simulink model "Sim"  (R2016a)
settings: Solver=VariableStepAuto  StartTime=0.0  StopTime=1500  FixedStep=1  RelTol=1e-3
values from neighbouring files (symbols this model uses):
  A = 7.841E16    (= 7.841e+16)    [Parameters.m]
  cv = 1820000    [Parameters.m]
  detaX = 0.0013333    [Parameters.m]
  Ea = 1.4766E5    (= 147660)    [Parameters.m]
  H_dr = 4.92E8    (= 492000000)    [Parameters.m]
  H_pc = 1.992E8    (= 199200000)    [Parameters.m]
  ord = 0.75    [Parameters.m]
  q_dot = 3.981E4    (= 39810)    [Parameters.m]
  T_0 = 298.15    [Parameters.m]
  Tl = 334.15    [Parameters.m]
  Ts = 331.15    [Parameters.m]
(part 2 of 3)

== system Sim/Element27 ==
  Q_in : Inport
  Q_out : Inport  Port=2
  Add : Sum  Inputs=++-
  Bias : Bias  Bias=1
  Bias2 : Bias  Bias=-Ts
  Bias3 : Bias  Bias=-Tl
  Bias4 : Bias  Bias=-1
  Constant : Constant  Value=cv+(H_pc/(Tl-Ts))
  Constant1 : Constant  Value=cv
  Constant2 : Constant  Value=0
  Constant3 : Constant  Value=ord
  Constant4 : Constant
  Divide : Product  Inputs=/
  Divide1 : Product  Inputs=/*
  Gain : Gain  Gain=-1
  Gain1 : Gain  Gain=(-8.314)/Ea
  Gain2 : Gain  Gain=(-1)*H_dr*A
  Gain3 : Gain  Gain=-1
  Gain4 : Gain  Gain=(-1)/H_dr
  Gain5 : Gain  Gain=1/(Tl-Ts)
  Gain6 : Gain  Gain=-1
  Integrator : Integrator  InitialCondition=T_0
  Integrator1 : Integrator
  Math Function : Math  SaturateOnIntegerOverflow=on
  Math Function1 : Math  Operator=pow  SaturateOnIntegerOverflow=on
  Product : Product
  Switch : Switch
  Switch1 : Switch  Criteria=u2 > Threshold
  Switch2 : Switch
  Switch3 : Switch  Criteria=u2 > Threshold
  Beta : Outport
  Temp : Outport  Port=2
  Alpha : Outport  Port=3
  wires:
  Q_out/1 -> Add/3
  Gain/1 -> Bias/1
  Divide1/1 -> Integrator/1  "dT/dt"
  Gain2/1 -> Product/1
  Integrator/1 -> Temp/1, Bias3/1, Bias2/1, Gain1/1  "T"
  Switch1/1 -> Divide1/1  "CON"
  Math Function1/1 -> Product/2
  Bias/1 -> Math Function1/1  "(1-Alpha)"
  Constant2/1 -> Switch2/3
  Add/1 -> Divide1/2  "CON*(dT/dt)"
  Gain5/1 -> Switch2/1, Switch2/2
  Switch2/1 -> Switch3/1, Bias4/1
  Constant/1 -> Switch/1
  Bias4/1 -> Gain6/1
  Switch/1 -> Switch1/1
  Switch3/1 -> Beta/1  "Beta"
  Gain6/1 -> Switch3/2
  Bias2/1 -> Gain5/1, Switch/2
  Constant4/1 -> Switch3/3
  Product/1 -> Add/1, Gain4/1  "-A*H_dr*exp()*(-Alhpa)"
  Gain1/1 -> Divide/1  "(-R*T)/Ea"
  Integrator1/1 -> Gain/1, Alpha/1  "Alpha"
  Gain4/1 -> Integrator1/1
  Constant3/1 -> Math Function1/2
  Constant1/1 -> Switch/3, Switch1/3
  Divide/1 -> Math Function/1  "Ea/(-R*T)"
  Math Function/1 -> Gain2/1
  Bias3/1 -> Gain3/1
  Gain3/1 -> Switch1/2
  Q_in/1 -> Add/2

== system Sim/Element28 ==
  Q_in : Inport
  Q_out : Inport  Port=2
  Add : Sum  Inputs=++-
  Bias : Bias  Bias=1
  Bias2 : Bias  Bias=-Ts
  Bias3 : Bias  Bias=-Tl
  Bias4 : Bias  Bias=-1
  Constant : Constant  Value=cv+(H_pc/(Tl-Ts))
  Constant1 : Constant  Value=cv
  Constant2 : Constant  Value=0
  Constant3 : Constant  Value=ord
  Constant4 : Constant
  Divide : Product  Inputs=/
  Divide1 : Product  Inputs=/*
  Gain : Gain  Gain=-1
  Gain1 : Gain  Gain=(-8.314)/Ea
  Gain2 : Gain  Gain=(-1)*H_dr*A
  Gain3 : Gain  Gain=-1
  Gain4 : Gain  Gain=(-1)/H_dr
  Gain5 : Gain  Gain=1/(Tl-Ts)
  Gain6 : Gain  Gain=-1
  Integrator : Integrator  InitialCondition=T_0
  Integrator1 : Integrator
  Math Function : Math  SaturateOnIntegerOverflow=on
  Math Function1 : Math  Operator=pow  SaturateOnIntegerOverflow=on
  Product : Product
  Switch : Switch
  Switch1 : Switch  Criteria=u2 > Threshold
  Switch2 : Switch
  Switch3 : Switch  Criteria=u2 > Threshold
  Beta : Outport
  Temp : Outport  Port=2
  Alpha : Outport  Port=3
  wires:
  Q_out/1 -> Add/3
  Gain/1 -> Bias/1
  Divide1/1 -> Integrator/1  "dT/dt"
  Gain2/1 -> Product/1
  Integrator/1 -> Temp/1, Bias3/1, Bias2/1, Gain1/1  "T"
  Switch1/1 -> Divide1/1  "CON"
  Math Function1/1 -> Product/2
  Bias/1 -> Math Function1/1  "(1-Alpha)"
  Constant2/1 -> Switch2/3
  Add/1 -> Divide1/2  "CON*(dT/dt)"
  Gain5/1 -> Switch2/1, Switch2/2
  Switch2/1 -> Switch3/1, Bias4/1
  Constant/1 -> Switch/1
  Bias4/1 -> Gain6/1
  Switch/1 -> Switch1/1
  Switch3/1 -> Beta/1  "Beta"
  Gain6/1 -> Switch3/2
  Bias2/1 -> Gain5/1, Switch/2
  Constant4/1 -> Switch3/3
  Product/1 -> Add/1, Gain4/1  "-A*H_dr*exp()*(-Alhpa)"
  Gain1/1 -> Divide/1  "(-R*T)/Ea"
  Integrator1/1 -> Gain/1, Alpha/1  "Alpha"
  Gain4/1 -> Integrator1/1
  Constant3/1 -> Math Function1/2
  Constant1/1 -> Switch/3, Switch1/3
  Divide/1 -> Math Function/1  "Ea/(-R*T)"
  Math Function/1 -> Gain2/1
  Bias3/1 -> Gain3/1
  Gain3/1 -> Switch1/2
  Q_in/1 -> Add/2

== system Sim/Element29 ==
  Q_in : Inport
  Q_out : Inport  Port=2
  Add : Sum  Inputs=++-
  Bias : Bias  Bias=1
  Bias2 : Bias  Bias=-Ts
  Bias3 : Bias  Bias=-Tl
  Bias4 : Bias  Bias=-1
  Constant : Constant  Value=cv+(H_pc/(Tl-Ts))
  Constant1 : Constant  Value=cv
  Constant2 : Constant  Value=0
  Constant3 : Constant  Value=ord
  Constant4 : Constant
  Divide : Product  Inputs=/
  Divide1 : Product  Inputs=/*
  Gain : Gain  Gain=-1
  Gain1 : Gain  Gain=(-8.314)/Ea
  Gain2 : Gain  Gain=(-1)*H_dr*A
  Gain3 : Gain  Gain=-1
  Gain4 : Gain  Gain=(-1)/H_dr
  Gain5 : Gain  Gain=1/(Tl-Ts)
  Gain6 : Gain  Gain=-1
  Integrator : Integrator  InitialCondition=T_0
  Integrator1 : Integrator
  Math Function : Math  SaturateOnIntegerOverflow=on
  Math Function1 : Math  Operator=pow  SaturateOnIntegerOverflow=on
  Product : Product
  Switch : Switch
  Switch1 : Switch  Criteria=u2 > Threshold
  Switch2 : Switch
  Switch3 : Switch  Criteria=u2 > Threshold
  Beta : Outport
  Temp : Outport  Port=2
  Alpha : Outport  Port=3
  wires:
  Q_out/1 -> Add/3
  Gain/1 -> Bias/1
  Divide1/1 -> Integrator/1  "dT/dt"
  Gain2/1 -> Product/1
  Integrator/1 -> Temp/1, Bias3/1, Bias2/1, Gain1/1  "T"
  Switch1/1 -> Divide1/1  "CON"
  Math Function1/1 -> Product/2
  Bias/1 -> Math Function1/1  "(1-Alpha)"
  Constant2/1 -> Switch2/3
  Add/1 -> Divide1/2  "CON*(dT/dt)"
  Gain5/1 -> Switch2/1, Switch2/2
  Switch2/1 -> Switch3/1, Bias4/1
  Constant/1 -> Switch/1
  Bias4/1 -> Gain6/1
  Switch/1 -> Switch1/1
  Switch3/1 -> Beta/1  "Beta"
  Gain6/1 -> Switch3/2
  Bias2/1 -> Gain5/1, Switch/2
  Constant4/1 -> Switch3/3
  Product/1 -> Add/1, Gain4/1  "-A*H_dr*exp()*(-Alhpa)"
  Gain1/1 -> Divide/1  "(-R*T)/Ea"
  Integrator1/1 -> Gain/1, Alpha/1  "Alpha"
  Gain4/1 -> Integrator1/1
  Constant3/1 -> Math Function1/2
  Constant1/1 -> Switch/3, Switch1/3
  Divide/1 -> Math Function/1  "Ea/(-R*T)"
  Math Function/1 -> Gain2/1
  Bias3/1 -> Gain3/1
  Gain3/1 -> Switch1/2
  Q_in/1 -> Add/2

== system Sim/Element3 ==
  Q_in : Inport
  Q_out : Inport  Port=2
  Add : Sum  Inputs=++-
  Bias : Bias  Bias=1
  Bias2 : Bias  Bias=-Ts
  Bias3 : Bias  Bias=-Tl
  Bias4 : Bias  Bias=-1
  Constant : Constant  Value=cv+(H_pc/(Tl-Ts))
  Constant1 : Constant  Value=cv
  Constant2 : Constant  Value=0
  Constant3 : Constant  Value=ord
  Constant4 : Constant
  Divide : Product  Inputs=/
  Divide1 : Product  Inputs=/*
  Gain : Gain  Gain=-1
  Gain1 : Gain  Gain=(-8.314)/Ea
  Gain2 : Gain  Gain=(-1)*H_dr*A
  Gain3 : Gain  Gain=-1
  Gain4 : Gain  Gain=(-1)/H_dr
  Gain5 : Gain  Gain=1/(Tl-Ts)
  Gain6 : Gain  Gain=-1
  Integrator : Integrator  InitialCondition=T_0
  Integrator1 : Integrator
  Math Function : Math  SaturateOnIntegerOverflow=on
  Math Function1 : Math  Operator=pow  SaturateOnIntegerOverflow=on
  Product : Product
  Switch : Switch
  Switch1 : Switch  Criteria=u2 > Threshold
  Switch2 : Switch
  Switch3 : Switch  Criteria=u2 > Threshold
  Beta : Outport
  Temp : Outport  Port=2
  Alpha : Outport  Port=3
  wires:
  Q_out/1 -> Add/3
  Gain/1 -> Bias/1
  Divide1/1 -> Integrator/1  "dT/dt"
  Gain2/1 -> Product/1
  Integrator/1 -> Temp/1, Bias3/1, Bias2/1, Gain1/1  "T"
  Switch1/1 -> Divide1/1  "CON"
  Math Function1/1 -> Product/2
  Bias/1 -> Math Function1/1  "(1-Alpha)"
  Constant2/1 -> Switch2/3
  Add/1 -> Divide1/2  "CON*(dT/dt)"
  Gain5/1 -> Switch2/1, Switch2/2
  Switch2/1 -> Switch3/1, Bias4/1
  Constant/1 -> Switch/1
  Bias4/1 -> Gain6/1
  Switch/1 -> Switch1/1
  Switch3/1 -> Beta/1  "Beta"
  Gain6/1 -> Switch3/2
  Bias2/1 -> Gain5/1, Switch/2
  Constant4/1 -> Switch3/3
  Product/1 -> Add/1, Gain4/1  "-A*H_dr*exp()*(-Alhpa)"
  Gain1/1 -> Divide/1  "(-R*T)/Ea"
  Integrator1/1 -> Gain/1, Alpha/1  "Alpha"
  Gain4/1 -> Integrator1/1
  Constant3/1 -> Math Function1/2
  Constant1/1 -> Switch/3, Switch1/3
  Divide/1 -> Math Function/1  "Ea/(-R*T)"
  Math Function/1 -> Gain2/1
  Bias3/1 -> Gain3/1
  Gain3/1 -> Switch1/2
  Q_in/1 -> Add/2

== system Sim/Element30 ==
  Q_in : Inport
  Q_out : Inport  Port=2
  Add : Sum  Inputs=++-
  Bias : Bias  Bias=1
  Bias2 : Bias  Bias=-Ts
  Bias3 : Bias  Bias=-Tl
  Bias4 : Bias  Bias=-1
  Constant : Constant  Value=cv+(H_pc/(Tl-Ts))
  Constant1 : Constant  Value=cv
  Constant2 : Constant  Value=0
  Constant3 : Constant  Value=ord
  Constant4 : Constant
  Divide : Product  Inputs=/
  Divide1 : Product  Inputs=/*
  Gain : Gain  Gain=-1
  Gain1 : Gain  Gain=(-8.314)/Ea
  Gain2 : Gain  Gain=(-1)*H_dr*A
  Gain3 : Gain  Gain=-1
  Gain4 : Gain  Gain=(-1)/H_dr
  Gain5 : Gain  Gain=1/(Tl-Ts)
  Gain6 : Gain  Gain=-1
  Integrator : Integrator  InitialCondition=T_0
  Integrator1 : Integrator
  Math Function : Math  SaturateOnIntegerOverflow=on
  Math Function1 : Math  Operator=pow  SaturateOnIntegerOverflow=on
  Product : Product
  Switch : Switch
  Switch1 : Switch  Criteria=u2 > Threshold
  Switch2 : Switch
  Switch3 : Switch  Criteria=u2 > Threshold
  Beta : Outport
  Temp : Outport  Port=2
  Alpha : Outport  Port=3
  wires:
  Q_out/1 -> Add/3
  Gain/1 -> Bias/1
  Divide1/1 -> Integrator/1  "dT/dt"
  Gain2/1 -> Product/1
  Integrator/1 -> Temp/1, Bias3/1, Bias2/1, Gain1/1  "T"
  Switch1/1 -> Divide1/1  "CON"
  Math Function1/1 -> Product/2
  Bias/1 -> Math Function1/1  "(1-Alpha)"
  Constant2/1 -> Switch2/3
  Add/1 -> Divide1/2  "CON*(dT/dt)"
  Gain5/1 -> Switch2/1, Switch2/2
  Switch2/1 -> Switch3/1, Bias4/1
  Constant/1 -> Switch/1
  Bias4/1 -> Gain6/1
  Switch/1 -> Switch1/1
  Switch3/1 -> Beta/1  "Beta"
  Gain6/1 -> Switch3/2
  Bias2/1 -> Gain5/1, Switch/2
  Constant4/1 -> Switch3/3
  Product/1 -> Add/1, Gain4/1  "-A*H_dr*exp()*(-Alhpa)"
  Gain1/1 -> Divide/1  "(-R*T)/Ea"
  Integrator1/1 -> Gain/1, Alpha/1  "Alpha"
  Gain4/1 -> Integrator1/1
  Constant3/1 -> Math Function1/2
  Constant1/1 -> Switch/3, Switch1/3
  Divide/1 -> Math Function/1  "Ea/(-R*T)"
  Math Function/1 -> Gain2/1
  Bias3/1 -> Gain3/1
  Gain3/1 -> Switch1/2
  Q_in/1 -> Add/2

== system Sim/Element31 ==
  Q_in : Inport
  Q_out : Inport  Port=2
  Add : Sum  Inputs=++-
  Bias : Bias  Bias=1
  Bias2 : Bias  Bias=-Ts
  Bias3 : Bias  Bias=-Tl
  Bias4 : Bias  Bias=-1
  Constant : Constant  Value=cv+(H_pc/(Tl-Ts))
  Constant1 : Constant  Value=cv
  Constant2 : Constant  Value=0
  Constant3 : Constant  Value=ord
  Constant4 : Constant
  Divide : Product  Inputs=/
  Divide1 : Product  Inputs=/*
  Gain : Gain  Gain=-1
  Gain1 : Gain  Gain=(-8.314)/Ea
  Gain2 : Gain  Gain=(-1)*H_dr*A
  Gain3 : Gain  Gain=-1
  Gain4 : Gain  Gain=(-1)/H_dr
  Gain5 : Gain  Gain=1/(Tl-Ts)
  Gain6 : Gain  Gain=-1
  Integrator : Integrator  InitialCondition=T_0
  Integrator1 : Integrator
  Math Function : Math  SaturateOnIntegerOverflow=on
  Math Function1 : Math  Operator=pow  SaturateOnIntegerOverflow=on
  Product : Product
  Switch : Switch
  Switch1 : Switch  Criteria=u2 > Threshold
  Switch2 : Switch
  Switch3 : Switch  Criteria=u2 > Threshold
  Beta : Outport
  Temp : Outport  Port=2
  Alpha : Outport  Port=3
  wires:
  Q_out/1 -> Add/3
  Gain/1 -> Bias/1
  Divide1/1 -> Integrator/1  "dT/dt"
  Gain2/1 -> Product/1
  Integrator/1 -> Temp/1, Bias3/1, Bias2/1, Gain1/1  "T"
  Switch1/1 -> Divide1/1  "CON"
  Math Function1/1 -> Product/2
  Bias/1 -> Math Function1/1  "(1-Alpha)"
  Constant2/1 -> Switch2/3
  Add/1 -> Divide1/2  "CON*(dT/dt)"
  Gain5/1 -> Switch2/1, Switch2/2
  Switch2/1 -> Switch3/1, Bias4/1
  Constant/1 -> Switch/1
  Bias4/1 -> Gain6/1
  Switch/1 -> Switch1/1
  Switch3/1 -> Beta/1  "Beta"
  Gain6/1 -> Switch3/2
  Bias2/1 -> Gain5/1, Switch/2
  Constant4/1 -> Switch3/3
  Product/1 -> Add/1, Gain4/1  "-A*H_dr*exp()*(-Alhpa)"
  Gain1/1 -> Divide/1  "(-R*T)/Ea"
  Integrator1/1 -> Gain/1, Alpha/1  "Alpha"
  Gain4/1 -> Integrator1/1
  Constant3/1 -> Math Function1/2
  Constant1/1 -> Switch/3, Switch1/3
  Divide/1 -> Math Function/1  "Ea/(-R*T)"
  Math Function/1 -> Gain2/1
  Bias3/1 -> Gain3/1
  Gain3/1 -> Switch1/2
  Q_in/1 -> Add/2

== system Sim/Element32 ==
  Q_in : Inport
  Q_out : Inport  Port=2
  Add : Sum  Inputs=++-
  Bias : Bias  Bias=1
  Bias2 : Bias  Bias=-Ts
  Bias3 : Bias  Bias=-Tl
  Bias4 : Bias  Bias=-1
  Constant : Constant  Value=cv+(H_pc/(Tl-Ts))
  Constant1 : Constant  Value=cv
  Constant2 : Constant  Value=0
  Constant3 : Constant  Value=ord
  Constant4 : Constant
  Divide : Product  Inputs=/
  Divide1 : Product  Inputs=/*
  Gain : Gain  Gain=-1
  Gain1 : Gain  Gain=(-8.314)/Ea
  Gain2 : Gain  Gain=(-1)*H_dr*A
  Gain3 : Gain  Gain=-1
  Gain4 : Gain  Gain=(-1)/H_dr
  Gain5 : Gain  Gain=1/(Tl-Ts)
  Gain6 : Gain  Gain=-1
  Integrator : Integrator  InitialCondition=T_0
  Integrator1 : Integrator
  Math Function : Math  SaturateOnIntegerOverflow=on
  Math Function1 : Math  Operator=pow  SaturateOnIntegerOverflow=on
  Product : Product
  Switch : Switch
  Switch1 : Switch  Criteria=u2 > Threshold
  Switch2 : Switch
  Switch3 : Switch  Criteria=u2 > Threshold
  Beta : Outport
  Temp : Outport  Port=2
  Alpha : Outport  Port=3
  wires:
  Q_out/1 -> Add/3
  Gain/1 -> Bias/1
  Divide1/1 -> Integrator/1  "dT/dt"
  Gain2/1 -> Product/1
  Integrator/1 -> Temp/1, Bias3/1, Bias2/1, Gain1/1  "T"
  Switch1/1 -> Divide1/1  "CON"
  Math Function1/1 -> Product/2
  Bias/1 -> Math Function1/1  "(1-Alpha)"
  Constant2/1 -> Switch2/3
  Add/1 -> Divide1/2  "CON*(dT/dt)"
  Gain5/1 -> Switch2/1, Switch2/2
  Switch2/1 -> Switch3/1, Bias4/1
  Constant/1 -> Switch/1
  Bias4/1 -> Gain6/1
  Switch/1 -> Switch1/1
  Switch3/1 -> Beta/1  "Beta"
  Gain6/1 -> Switch3/2
  Bias2/1 -> Gain5/1, Switch/2
  Constant4/1 -> Switch3/3
  Product/1 -> Add/1, Gain4/1  "-A*H_dr*exp()*(-Alhpa)"
  Gain1/1 -> Divide/1  "(-R*T)/Ea"
  Integrator1/1 -> Gain/1, Alpha/1  "Alpha"
  Gain4/1 -> Integrator1/1
  Constant3/1 -> Math Function1/2
  Constant1/1 -> Switch/3, Switch1/3
  Divide/1 -> Math Function/1  "Ea/(-R*T)"
  Math Function/1 -> Gain2/1
  Bias3/1 -> Gain3/1
  Gain3/1 -> Switch1/2
  Q_in/1 -> Add/2

== system Sim/Element33 ==
  Q_in : Inport
  Q_out : Inport  Port=2
  Add : Sum  Inputs=++-
  Bias : Bias  Bias=1
  Bias2 : Bias  Bias=-Ts
  Bias3 : Bias  Bias=-Tl
  Bias4 : Bias  Bias=-1
  Constant : Constant  Value=cv+(H_pc/(Tl-Ts))
  Constant1 : Constant  Value=cv
  Constant2 : Constant  Value=0
  Constant3 : Constant  Value=ord
  Constant4 : Constant
  Divide : Product  Inputs=/
  Divide1 : Product  Inputs=/*
  Gain : Gain  Gain=-1
  Gain1 : Gain  Gain=(-8.314)/Ea
  Gain2 : Gain  Gain=(-1)*H_dr*A
  Gain3 : Gain  Gain=-1
  Gain4 : Gain  Gain=(-1)/H_dr
  Gain5 : Gain  Gain=1/(Tl-Ts)
  Gain6 : Gain  Gain=-1
  Integrator : Integrator  InitialCondition=T_0
  Integrator1 : Integrator
  Math Function : Math  SaturateOnIntegerOverflow=on
  Math Function1 : Math  Operator=pow  SaturateOnIntegerOverflow=on
  Product : Product
  Switch : Switch
  Switch1 : Switch  Criteria=u2 > Threshold
  Switch2 : Switch
  Switch3 : Switch  Criteria=u2 > Threshold
  Beta : Outport
  Temp : Outport  Port=2
  Alpha : Outport  Port=3
  wires:
  Q_out/1 -> Add/3
  Gain/1 -> Bias/1
  Divide1/1 -> Integrator/1  "dT/dt"
  Gain2/1 -> Product/1
  Integrator/1 -> Temp/1, Bias3/1, Bias2/1, Gain1/1  "T"
  Switch1/1 -> Divide1/1  "CON"
  Math Function1/1 -> Product/2
  Bias/1 -> Math Function1/1  "(1-Alpha)"
  Constant2/1 -> Switch2/3
  Add/1 -> Divide1/2  "CON*(dT/dt)"
  Gain5/1 -> Switch2/1, Switch2/2
  Switch2/1 -> Switch3/1, Bias4/1
  Constant/1 -> Switch/1
  Bias4/1 -> Gain6/1
  Switch/1 -> Switch1/1
  Switch3/1 -> Beta/1  "Beta"
  Gain6/1 -> Switch3/2
  Bias2/1 -> Gain5/1, Switch/2
  Constant4/1 -> Switch3/3
  Product/1 -> Add/1, Gain4/1  "-A*H_dr*exp()*(-Alhpa)"
  Gain1/1 -> Divide/1  "(-R*T)/Ea"
  Integrator1/1 -> Gain/1, Alpha/1  "Alpha"
  Gain4/1 -> Integrator1/1
  Constant3/1 -> Math Function1/2
  Constant1/1 -> Switch/3, Switch1/3
  Divide/1 -> Math Function/1  "Ea/(-R*T)"
  Math Function/1 -> Gain2/1
  Bias3/1 -> Gain3/1
  Gain3/1 -> Switch1/2
  Q_in/1 -> Add/2

== system Sim/Element34 ==
  Q_in : Inport
  Q_out : Inport  Port=2
  Add : Sum  Inputs=++-
  Bias : Bias  Bias=1
  Bias2 : Bias  Bias=-Ts
  Bias3 : Bias  Bias=-Tl
  Bias4 : Bias  Bias=-1
  Constant : Constant  Value=cv+(H_pc/(Tl-Ts))
  Constant1 : Constant  Value=cv
  Constant2 : Constant  Value=0
  Constant3 : Constant  Value=ord
  Constant4 : Constant
  Divide : Product  Inputs=/
  Divide1 : Product  Inputs=/*
  Gain : Gain  Gain=-1
  Gain1 : Gain  Gain=(-8.314)/Ea
  Gain2 : Gain  Gain=(-1)*H_dr*A
  Gain3 : Gain  Gain=-1
  Gain4 : Gain  Gain=(-1)/H_dr
  Gain5 : Gain  Gain=1/(Tl-Ts)
  Gain6 : Gain  Gain=-1
  Integrator : Integrator  InitialCondition=T_0
  Integrator1 : Integrator
  Math Function : Math  SaturateOnIntegerOverflow=on
  Math Function1 : Math  Operator=pow  SaturateOnIntegerOverflow=on
  Product : Product
  Switch : Switch
  Switch1 : Switch  Criteria=u2 > Threshold
  Switch2 : Switch
  Switch3 : Switch  Criteria=u2 > Threshold
  Beta : Outport
  Temp : Outport  Port=2
  Alpha : Outport  Port=3
  wires:
  Q_out/1 -> Add/3
  Gain/1 -> Bias/1
  Divide1/1 -> Integrator/1  "dT/dt"
  Gain2/1 -> Product/1
  Integrator/1 -> Temp/1, Bias3/1, Bias2/1, Gain1/1  "T"
  Switch1/1 -> Divide1/1  "CON"
  Math Function1/1 -> Product/2
  Bias/1 -> Math Function1/1  "(1-Alpha)"
  Constant2/1 -> Switch2/3
  Add/1 -> Divide1/2  "CON*(dT/dt)"
  Gain5/1 -> Switch2/1, Switch2/2
  Switch2/1 -> Switch3/1, Bias4/1
  Constant/1 -> Switch/1
  Bias4/1 -> Gain6/1
  Switch/1 -> Switch1/1
  Switch3/1 -> Beta/1  "Beta"
  Gain6/1 -> Switch3/2
  Bias2/1 -> Gain5/1, Switch/2
  Constant4/1 -> Switch3/3
  Product/1 -> Add/1, Gain4/1  "-A*H_dr*exp()*(-Alhpa)"
  Gain1/1 -> Divide/1  "(-R*T)/Ea"
  Integrator1/1 -> Gain/1, Alpha/1  "Alpha"
  Gain4/1 -> Integrator1/1
  Constant3/1 -> Math Function1/2
  Constant1/1 -> Switch/3, Switch1/3
  Divide/1 -> Math Function/1  "Ea/(-R*T)"
  Math Function/1 -> Gain2/1
  Bias3/1 -> Gain3/1
  Gain3/1 -> Switch1/2
  Q_in/1 -> Add/2

== system Sim/Element35 ==
  Q_in : Inport
  Q_out : Inport  Port=2
  Add : Sum  Inputs=++-
  Bias : Bias  Bias=1
  Bias2 : Bias  Bias=-Ts
  Bias3 : Bias  Bias=-Tl
  Bias4 : Bias  Bias=-1
  Constant : Constant  Value=cv+(H_pc/(Tl-Ts))
  Constant1 : Constant  Value=cv
  Constant2 : Constant  Value=0
  Constant3 : Constant  Value=ord
  Constant4 : Constant
  Divide : Product  Inputs=/
  Divide1 : Product  Inputs=/*
  Gain : Gain  Gain=-1
  Gain1 : Gain  Gain=(-8.314)/Ea
  Gain2 : Gain  Gain=(-1)*H_dr*A
  Gain3 : Gain  Gain=-1
  Gain4 : Gain  Gain=(-1)/H_dr
  Gain5 : Gain  Gain=1/(Tl-Ts)
  Gain6 : Gain  Gain=-1
  Integrator : Integrator  InitialCondition=T_0
  Integrator1 : Integrator
  Math Function : Math  SaturateOnIntegerOverflow=on
  Math Function1 : Math  Operator=pow  SaturateOnIntegerOverflow=on
  Product : Product
  Switch : Switch
  Switch1 : Switch  Criteria=u2 > Threshold
  Switch2 : Switch
  Switch3 : Switch  Criteria=u2 > Threshold
  Beta : Outport
  Temp : Outport  Port=2
  Alpha : Outport  Port=3
  wires:
  Q_out/1 -> Add/3
  Gain/1 -> Bias/1
  Divide1/1 -> Integrator/1  "dT/dt"
  Gain2/1 -> Product/1
  Integrator/1 -> Temp/1, Bias3/1, Bias2/1, Gain1/1  "T"
  Switch1/1 -> Divide1/1  "CON"
  Math Function1/1 -> Product/2
  Bias/1 -> Math Function1/1  "(1-Alpha)"
  Constant2/1 -> Switch2/3
  Add/1 -> Divide1/2  "CON*(dT/dt)"
  Gain5/1 -> Switch2/1, Switch2/2
  Switch2/1 -> Switch3/1, Bias4/1
  Constant/1 -> Switch/1
  Bias4/1 -> Gain6/1
  Switch/1 -> Switch1/1
  Switch3/1 -> Beta/1  "Beta"
  Gain6/1 -> Switch3/2
  Bias2/1 -> Gain5/1, Switch/2
  Constant4/1 -> Switch3/3
  Product/1 -> Add/1, Gain4/1  "-A*H_dr*exp()*(-Alhpa)"
  Gain1/1 -> Divide/1  "(-R*T)/Ea"
  Integrator1/1 -> Gain/1, Alpha/1  "Alpha"
  Gain4/1 -> Integrator1/1
  Constant3/1 -> Math Function1/2
  Constant1/1 -> Switch/3, Switch1/3
  Divide/1 -> Math Function/1  "Ea/(-R*T)"
  Math Function/1 -> Gain2/1
  Bias3/1 -> Gain3/1
  Gain3/1 -> Switch1/2
  Q_in/1 -> Add/2

== system Sim/Element36 ==
  Q_in : Inport
  Q_out : Inport  Port=2
  Add : Sum  Inputs=++-
  Bias : Bias  Bias=1
  Bias2 : Bias  Bias=-Ts
  Bias3 : Bias  Bias=-Tl
  Bias4 : Bias  Bias=-1
  Constant : Constant  Value=cv+(H_pc/(Tl-Ts))
  Constant1 : Constant  Value=cv
  Constant2 : Constant  Value=0
  Constant3 : Constant  Value=ord
  Constant4 : Constant
  Divide : Product  Inputs=/
  Divide1 : Product  Inputs=/*
  Gain : Gain  Gain=-1
  Gain1 : Gain  Gain=(-8.314)/Ea
  Gain2 : Gain  Gain=(-1)*H_dr*A
  Gain3 : Gain  Gain=-1
  Gain4 : Gain  Gain=(-1)/H_dr
  Gain5 : Gain  Gain=1/(Tl-Ts)
  Gain6 : Gain  Gain=-1
  Integrator : Integrator  InitialCondition=T_0
  Integrator1 : Integrator
  Math Function : Math  SaturateOnIntegerOverflow=on
  Math Function1 : Math  Operator=pow  SaturateOnIntegerOverflow=on
  Product : Product
  Switch : Switch
  Switch1 : Switch  Criteria=u2 > Threshold
  Switch2 : Switch
  Switch3 : Switch  Criteria=u2 > Threshold
  Beta : Outport
  Temp : Outport  Port=2
  Alpha : Outport  Port=3
  wires:
  Q_out/1 -> Add/3
  Gain/1 -> Bias/1
  Divide1/1 -> Integrator/1  "dT/dt"
  Gain2/1 -> Product/1
  Integrator/1 -> Temp/1, Bias3/1, Bias2/1, Gain1/1  "T"
  Switch1/1 -> Divide1/1  "CON"
  Math Function1/1 -> Product/2
  Bias/1 -> Math Function1/1  "(1-Alpha)"
  Constant2/1 -> Switch2/3
  Add/1 -> Divide1/2  "CON*(dT/dt)"
  Gain5/1 -> Switch2/1, Switch2/2
  Switch2/1 -> Switch3/1, Bias4/1
  Constant/1 -> Switch/1
  Bias4/1 -> Gain6/1
  Switch/1 -> Switch1/1
  Switch3/1 -> Beta/1  "Beta"
  Gain6/1 -> Switch3/2
  Bias2/1 -> Gain5/1, Switch/2
  Constant4/1 -> Switch3/3
  Product/1 -> Add/1, Gain4/1  "-A*H_dr*exp()*(-Alhpa)"
  Gain1/1 -> Divide/1  "(-R*T)/Ea"
  Integrator1/1 -> Gain/1, Alpha/1  "Alpha"
  Gain4/1 -> Integrator1/1
  Constant3/1 -> Math Function1/2
  Constant1/1 -> Switch/3, Switch1/3
  Divide/1 -> Math Function/1  "Ea/(-R*T)"
  Math Function/1 -> Gain2/1
  Bias3/1 -> Gain3/1
  Gain3/1 -> Switch1/2
  Q_in/1 -> Add/2

== system Sim/Element37 ==
  Q_in : Inport
  Q_out : Inport  Port=2
  Add : Sum  Inputs=++-
  Bias : Bias  Bias=1
  Bias2 : Bias  Bias=-Ts
  Bias3 : Bias  Bias=-Tl
  Bias4 : Bias  Bias=-1
  Constant : Constant  Value=cv+(H_pc/(Tl-Ts))
  Constant1 : Constant  Value=cv
  Constant2 : Constant  Value=0
  Constant3 : Constant  Value=ord
  Constant4 : Constant
  Divide : Product  Inputs=/
  Divide1 : Product  Inputs=/*
  Gain : Gain  Gain=-1
  Gain1 : Gain  Gain=(-8.314)/Ea
  Gain2 : Gain  Gain=(-1)*H_dr*A
  Gain3 : Gain  Gain=-1
  Gain4 : Gain  Gain=(-1)/H_dr
  Gain5 : Gain  Gain=1/(Tl-Ts)
  Gain6 : Gain  Gain=-1
  Integrator : Integrator  InitialCondition=T_0
  Integrator1 : Integrator
  Math Function : Math  SaturateOnIntegerOverflow=on
  Math Function1 : Math  Operator=pow  SaturateOnIntegerOverflow=on
  Product : Product
  Switch : Switch
  Switch1 : Switch  Criteria=u2 > Threshold
  Switch2 : Switch
  Switch3 : Switch  Criteria=u2 > Threshold
  Beta : Outport
  Temp : Outport  Port=2
  Alpha : Outport  Port=3
  wires:
  Q_out/1 -> Add/3
  Gain/1 -> Bias/1
  Divide1/1 -> Integrator/1  "dT/dt"
  Gain2/1 -> Product/1
  Integrator/1 -> Temp/1, Bias3/1, Bias2/1, Gain1/1  "T"
  Switch1/1 -> Divide1/1  "CON"
  Math Function1/1 -> Product/2
  Bias/1 -> Math Function1/1  "(1-Alpha)"
  Constant2/1 -> Switch2/3
  Add/1 -> Divide1/2  "CON*(dT/dt)"
  Gain5/1 -> Switch2/1, Switch2/2
  Switch2/1 -> Switch3/1, Bias4/1
  Constant/1 -> Switch/1
  Bias4/1 -> Gain6/1
  Switch/1 -> Switch1/1
  Switch3/1 -> Beta/1  "Beta"
  Gain6/1 -> Switch3/2
  Bias2/1 -> Gain5/1, Switch/2
  Constant4/1 -> Switch3/3
  Product/1 -> Add/1, Gain4/1  "-A*H_dr*exp()*(-Alhpa)"
  Gain1/1 -> Divide/1  "(-R*T)/Ea"
  Integrator1/1 -> Gain/1, Alpha/1  "Alpha"
  Gain4/1 -> Integrator1/1
  Constant3/1 -> Math Function1/2
  Constant1/1 -> Switch/3, Switch1/3
  Divide/1 -> Math Function/1  "Ea/(-R*T)"
  Math Function/1 -> Gain2/1
  Bias3/1 -> Gain3/1
  Gain3/1 -> Switch1/2
  Q_in/1 -> Add/2

== system Sim/Element38 ==
  Q_in : Inport
  Q_out : Inport  Port=2
  Add : Sum  Inputs=++-
  Bias : Bias  Bias=1
  Bias2 : Bias  Bias=-Ts
  Bias3 : Bias  Bias=-Tl
  Bias4 : Bias  Bias=-1
  Constant : Constant  Value=cv+(H_pc/(Tl-Ts))
  Constant1 : Constant  Value=cv
  Constant2 : Constant  Value=0
  Constant3 : Constant  Value=ord
  Constant4 : Constant
  Divide : Product  Inputs=/
  Divide1 : Product  Inputs=/*
  Gain : Gain  Gain=-1
  Gain1 : Gain  Gain=(-8.314)/Ea
  Gain2 : Gain  Gain=(-1)*H_dr*A
  Gain3 : Gain  Gain=-1
  Gain4 : Gain  Gain=(-1)/H_dr
  Gain5 : Gain  Gain=1/(Tl-Ts)
  Gain6 : Gain  Gain=-1
  Integrator : Integrator  InitialCondition=T_0
  Integrator1 : Integrator
  Math Function : Math  SaturateOnIntegerOverflow=on
  Math Function1 : Math  Operator=pow  SaturateOnIntegerOverflow=on
  Product : Product
  Switch : Switch
  Switch1 : Switch  Criteria=u2 > Threshold
  Switch2 : Switch
  Switch3 : Switch  Criteria=u2 > Threshold
  Beta : Outport
  Temp : Outport  Port=2
  Alpha : Outport  Port=3
  wires:
  Q_out/1 -> Add/3
  Gain/1 -> Bias/1
  Divide1/1 -> Integrator/1  "dT/dt"
  Gain2/1 -> Product/1
  Integrator/1 -> Temp/1, Bias3/1, Bias2/1, Gain1/1  "T"
  Switch1/1 -> Divide1/1  "CON"
  Math Function1/1 -> Product/2
  Bias/1 -> Math Function1/1  "(1-Alpha)"
  Constant2/1 -> Switch2/3
  Add/1 -> Divide1/2  "CON*(dT/dt)"
  Gain5/1 -> Switch2/1, Switch2/2
  Switch2/1 -> Switch3/1, Bias4/1
  Constant/1 -> Switch/1
  Bias4/1 -> Gain6/1
  Switch/1 -> Switch1/1
  Switch3/1 -> Beta/1  "Beta"
  Gain6/1 -> Switch3/2
  Bias2/1 -> Gain5/1, Switch/2
  Constant4/1 -> Switch3/3
  Product/1 -> Add/1, Gain4/1  "-A*H_dr*exp()*(-Alhpa)"
  Gain1/1 -> Divide/1  "(-R*T)/Ea"
  Integrator1/1 -> Gain/1, Alpha/1  "Alpha"
  Gain4/1 -> Integrator1/1
  Constant3/1 -> Math Function1/2
  Constant1/1 -> Switch/3, Switch1/3
  Divide/1 -> Math Function/1  "Ea/(-R*T)"
  Math Function/1 -> Gain2/1
  Bias3/1 -> Gain3/1
  Gain3/1 -> Switch1/2
  Q_in/1 -> Add/2

== system Sim/Element39 ==
  Q_in : Inport
  Q_out : Inport  Port=2
  Add : Sum  Inputs=++-
  Bias : Bias  Bias=1
  Bias2 : Bias  Bias=-Ts
  Bias3 : Bias  Bias=-Tl
  Bias4 : Bias  Bias=-1
  Constant : Constant  Value=cv+(H_pc/(Tl-Ts))
  Constant1 : Constant  Value=cv
  Constant2 : Constant  Value=0
  Constant3 : Constant  Value=ord
  Constant4 : Constant
  Divide : Product  Inputs=/
  Divide1 : Product  Inputs=/*
  Gain : Gain  Gain=-1
  Gain1 : Gain  Gain=(-8.314)/Ea
  Gain2 : Gain  Gain=(-1)*H_dr*A
  Gain3 : Gain  Gain=-1
  Gain4 : Gain  Gain=(-1)/H_dr
  Gain5 : Gain  Gain=1/(Tl-Ts)
  Gain6 : Gain  Gain=-1
  Integrator : Integrator  InitialCondition=T_0
  Integrator1 : Integrator
  Math Function : Math  SaturateOnIntegerOverflow=on
  Math Function1 : Math  Operator=pow  SaturateOnIntegerOverflow=on
  Product : Product
  Switch : Switch
  Switch1 : Switch  Criteria=u2 > Threshold
  Switch2 : Switch
  Switch3 : Switch  Criteria=u2 > Threshold
  Beta : Outport
  Temp : Outport  Port=2
  Alpha : Outport  Port=3
  wires:
  Q_out/1 -> Add/3
  Gain/1 -> Bias/1
  Divide1/1 -> Integrator/1  "dT/dt"
  Gain2/1 -> Product/1
  Integrator/1 -> Temp/1, Bias3/1, Bias2/1, Gain1/1  "T"
  Switch1/1 -> Divide1/1  "CON"
  Math Function1/1 -> Product/2
  Bias/1 -> Math Function1/1  "(1-Alpha)"
  Constant2/1 -> Switch2/3
  Add/1 -> Divide1/2  "CON*(dT/dt)"
  Gain5/1 -> Switch2/1, Switch2/2
  Switch2/1 -> Switch3/1, Bias4/1
  Constant/1 -> Switch/1
  Bias4/1 -> Gain6/1
  Switch/1 -> Switch1/1
  Switch3/1 -> Beta/1  "Beta"
  Gain6/1 -> Switch3/2
  Bias2/1 -> Gain5/1, Switch/2
  Constant4/1 -> Switch3/3
  Product/1 -> Add/1, Gain4/1  "-A*H_dr*exp()*(-Alhpa)"
  Gain1/1 -> Divide/1  "(-R*T)/Ea"
  Integrator1/1 -> Gain/1, Alpha/1  "Alpha"
  Gain4/1 -> Integrator1/1
  Constant3/1 -> Math Function1/2
  Constant1/1 -> Switch/3, Switch1/3
  Divide/1 -> Math Function/1  "Ea/(-R*T)"
  Math Function/1 -> Gain2/1
  Bias3/1 -> Gain3/1
  Gain3/1 -> Switch1/2
  Q_in/1 -> Add/2

== system Sim/Element4 ==
  Q_in : Inport
  Q_out : Inport  Port=2
  Add : Sum  Inputs=++-
  Bias : Bias  Bias=1
  Bias2 : Bias  Bias=-Ts
  Bias3 : Bias  Bias=-Tl
  Bias4 : Bias  Bias=-1
  Constant : Constant  Value=cv+(H_pc/(Tl-Ts))
  Constant1 : Constant  Value=cv
  Constant2 : Constant  Value=0
  Constant3 : Constant  Value=ord
  Constant4 : Constant
  Divide : Product  Inputs=/
  Divide1 : Product  Inputs=/*
  Gain : Gain  Gain=-1
  Gain1 : Gain  Gain=(-8.314)/Ea
  Gain2 : Gain  Gain=(-1)*H_dr*A
  Gain3 : Gain  Gain=-1
  Gain4 : Gain  Gain=(-1)/H_dr
  Gain5 : Gain  Gain=1/(Tl-Ts)
  Gain6 : Gain  Gain=-1
  Integrator : Integrator  InitialCondition=T_0
  Integrator1 : Integrator
  Math Function : Math  SaturateOnIntegerOverflow=on
  Math Function1 : Math  Operator=pow  SaturateOnIntegerOverflow=on
  Product : Product
  Switch : Switch
  Switch1 : Switch  Criteria=u2 > Threshold
  Switch2 : Switch
  Switch3 : Switch  Criteria=u2 > Threshold
  Beta : Outport
  Temp : Outport  Port=2
  Alpha : Outport  Port=3
  wires:
  Q_out/1 -> Add/3
  Gain/1 -> Bias/1
  Divide1/1 -> Integrator/1  "dT/dt"
  Gain2/1 -> Product/1
  Integrator/1 -> Temp/1, Bias3/1, Bias2/1, Gain1/1  "T"
  Switch1/1 -> Divide1/1  "CON"
  Math Function1/1 -> Product/2
  Bias/1 -> Math Function1/1  "(1-Alpha)"
  Constant2/1 -> Switch2/3
  Add/1 -> Divide1/2  "CON*(dT/dt)"
  Gain5/1 -> Switch2/1, Switch2/2
  Switch2/1 -> Switch3/1, Bias4/1
  Constant/1 -> Switch/1
  Bias4/1 -> Gain6/1
  Switch/1 -> Switch1/1
  Switch3/1 -> Beta/1  "Beta"
  Gain6/1 -> Switch3/2
  Bias2/1 -> Gain5/1, Switch/2
  Constant4/1 -> Switch3/3
  Product/1 -> Add/1, Gain4/1  "-A*H_dr*exp()*(-Alhpa)"
  Gain1/1 -> Divide/1  "(-R*T)/Ea"
  Integrator1/1 -> Gain/1, Alpha/1  "Alpha"
  Gain4/1 -> Integrator1/1
  Constant3/1 -> Math Function1/2
  Constant1/1 -> Switch/3, Switch1/3
  Divide/1 -> Math Function/1  "Ea/(-R*T)"
  Math Function/1 -> Gain2/1
  Bias3/1 -> Gain3/1
  Gain3/1 -> Switch1/2
  Q_in/1 -> Add/2

== system Sim/Element40 ==
  Q_in : Inport
  Q_out : Inport  Port=2
  Add : Sum  Inputs=++-
  Bias : Bias  Bias=1
  Bias2 : Bias  Bias=-Ts
  Bias3 : Bias  Bias=-Tl
  Bias4 : Bias  Bias=-1
  Constant : Constant  Value=cv+(H_pc/(Tl-Ts))
  Constant1 : Constant  Value=cv
  Constant2 : Constant  Value=0
  Constant3 : Constant  Value=ord
  Constant4 : Constant
  Divide : Product  Inputs=/
  Divide1 : Product  Inputs=/*
  Gain : Gain  Gain=-1
  Gain1 : Gain  Gain=(-8.314)/Ea
  Gain2 : Gain  Gain=(-1)*H_dr*A
  Gain3 : Gain  Gain=-1
  Gain4 : Gain  Gain=(-1)/H_dr
  Gain5 : Gain  Gain=1/(Tl-Ts)
  Gain6 : Gain  Gain=-1
  Integrator : Integrator  InitialCondition=T_0
  Integrator1 : Integrator
  Math Function : Math  SaturateOnIntegerOverflow=on
  Math Function1 : Math  Operator=pow  SaturateOnIntegerOverflow=on
  Product : Product
  Switch : Switch
  Switch1 : Switch  Criteria=u2 > Threshold
  Switch2 : Switch
  Switch3 : Switch  Criteria=u2 > Threshold
  Beta : Outport
  Temp : Outport  Port=2
  Alpha : Outport  Port=3
  wires:
  Q_out/1 -> Add/3
  Gain/1 -> Bias/1
  Divide1/1 -> Integrator/1  "dT/dt"
  Gain2/1 -> Product/1
  Integrator/1 -> Temp/1, Bias3/1, Bias2/1, Gain1/1  "T"
  Switch1/1 -> Divide1/1  "CON"
  Math Function1/1 -> Product/2
  Bias/1 -> Math Function1/1  "(1-Alpha)"
  Constant2/1 -> Switch2/3
  Add/1 -> Divide1/2  "CON*(dT/dt)"
  Gain5/1 -> Switch2/1, Switch2/2
  Switch2/1 -> Switch3/1, Bias4/1
  Constant/1 -> Switch/1
  Bias4/1 -> Gain6/1
  Switch/1 -> Switch1/1
  Switch3/1 -> Beta/1  "Beta"
  Gain6/1 -> Switch3/2
  Bias2/1 -> Gain5/1, Switch/2
  Constant4/1 -> Switch3/3
  Product/1 -> Add/1, Gain4/1  "-A*H_dr*exp()*(-Alhpa)"
  Gain1/1 -> Divide/1  "(-R*T)/Ea"
  Integrator1/1 -> Gain/1, Alpha/1  "Alpha"
  Gain4/1 -> Integrator1/1
  Constant3/1 -> Math Function1/2
  Constant1/1 -> Switch/3, Switch1/3
  Divide/1 -> Math Function/1  "Ea/(-R*T)"
  Math Function/1 -> Gain2/1
  Bias3/1 -> Gain3/1
  Gain3/1 -> Switch1/2
  Q_in/1 -> Add/2

== system Sim/Element41 ==
  Q_in : Inport
  Q_out : Inport  Port=2
  Add : Sum  Inputs=++-
  Bias : Bias  Bias=1
  Bias2 : Bias  Bias=-Ts
  Bias3 : Bias  Bias=-Tl
  Bias4 : Bias  Bias=-1
  Constant : Constant  Value=cv+(H_pc/(Tl-Ts))
  Constant1 : Constant  Value=cv
  Constant2 : Constant  Value=0
  Constant3 : Constant  Value=ord
  Constant4 : Constant
  Divide : Product  Inputs=/
  Divide1 : Product  Inputs=/*
  Gain : Gain  Gain=-1
  Gain1 : Gain  Gain=(-8.314)/Ea
  Gain2 : Gain  Gain=(-1)*H_dr*A
  Gain3 : Gain  Gain=-1
  Gain4 : Gain  Gain=(-1)/H_dr
  Gain5 : Gain  Gain=1/(Tl-Ts)
  Gain6 : Gain  Gain=-1
  Integrator : Integrator  InitialCondition=T_0
  Integrator1 : Integrator
  Math Function : Math  SaturateOnIntegerOverflow=on
  Math Function1 : Math  Operator=pow  SaturateOnIntegerOverflow=on
  Product : Product
  Switch : Switch
  Switch1 : Switch  Criteria=u2 > Threshold
  Switch2 : Switch
  Switch3 : Switch  Criteria=u2 > Threshold
  Beta : Outport
  Temp : Outport  Port=2
  Alpha : Outport  Port=3
  wires:
  Q_out/1 -> Add/3
  Gain/1 -> Bias/1
  Divide1/1 -> Integrator/1  "dT/dt"
  Gain2/1 -> Product/1
  Integrator/1 -> Temp/1, Bias3/1, Bias2/1, Gain1/1  "T"
  Switch1/1 -> Divide1/1  "CON"
  Math Function1/1 -> Product/2
  Bias/1 -> Math Function1/1  "(1-Alpha)"
  Constant2/1 -> Switch2/3
  Add/1 -> Divide1/2  "CON*(dT/dt)"
  Gain5/1 -> Switch2/1, Switch2/2
  Switch2/1 -> Switch3/1, Bias4/1
  Constant/1 -> Switch/1
  Bias4/1 -> Gain6/1
  Switch/1 -> Switch1/1
  Switch3/1 -> Beta/1  "Beta"
  Gain6/1 -> Switch3/2
  Bias2/1 -> Gain5/1, Switch/2
  Constant4/1 -> Switch3/3
  Product/1 -> Add/1, Gain4/1  "-A*H_dr*exp()*(-Alhpa)"
  Gain1/1 -> Divide/1  "(-R*T)/Ea"
  Integrator1/1 -> Gain/1, Alpha/1  "Alpha"
  Gain4/1 -> Integrator1/1
  Constant3/1 -> Math Function1/2
  Constant1/1 -> Switch/3, Switch1/3
  Divide/1 -> Math Function/1  "Ea/(-R*T)"
  Math Function/1 -> Gain2/1
  Bias3/1 -> Gain3/1
  Gain3/1 -> Switch1/2
  Q_in/1 -> Add/2

== system Sim/Element42 ==
  Q_in : Inport
  Q_out : Inport  Port=2
  Add : Sum  Inputs=++-
  Bias : Bias  Bias=1
  Bias2 : Bias  Bias=-Ts
  Bias3 : Bias  Bias=-Tl
  Bias4 : Bias  Bias=-1
  Constant : Constant  Value=cv+(H_pc/(Tl-Ts))
  Constant1 : Constant  Value=cv
  Constant2 : Constant  Value=0
  Constant3 : Constant  Value=ord
  Constant4 : Constant
  Divide : Product  Inputs=/
  Divide1 : Product  Inputs=/*
  Gain : Gain  Gain=-1
  Gain1 : Gain  Gain=(-8.314)/Ea
  Gain2 : Gain  Gain=(-1)*H_dr*A
  Gain3 : Gain  Gain=-1
  Gain4 : Gain  Gain=(-1)/H_dr
  Gain5 : Gain  Gain=1/(Tl-Ts)
  Gain6 : Gain  Gain=-1
  Integrator : Integrator  InitialCondition=T_0
  Integrator1 : Integrator
  Math Function : Math  SaturateOnIntegerOverflow=on
  Math Function1 : Math  Operator=pow  SaturateOnIntegerOverflow=on
  Product : Product
  Switch : Switch
  Switch1 : Switch  Criteria=u2 > Threshold
  Switch2 : Switch
  Switch3 : Switch  Criteria=u2 > Threshold
  Beta : Outport
  Temp : Outport  Port=2
  Alpha : Outport  Port=3
  wires:
  Q_out/1 -> Add/3
  Gain/1 -> Bias/1
  Divide1/1 -> Integrator/1  "dT/dt"
  Gain2/1 -> Product/1
  Integrator/1 -> Temp/1, Bias3/1, Bias2/1, Gain1/1  "T"
  Switch1/1 -> Divide1/1  "CON"
  Math Function1/1 -> Product/2
  Bias/1 -> Math Function1/1  "(1-Alpha)"
  Constant2/1 -> Switch2/3
  Add/1 -> Divide1/2  "CON*(dT/dt)"
  Gain5/1 -> Switch2/1, Switch2/2
  Switch2/1 -> Switch3/1, Bias4/1
  Constant/1 -> Switch/1
  Bias4/1 -> Gain6/1
  Switch/1 -> Switch1/1
  Switch3/1 -> Beta/1  "Beta"
  Gain6/1 -> Switch3/2
  Bias2/1 -> Gain5/1, Switch/2
  Constant4/1 -> Switch3/3
  Product/1 -> Add/1, Gain4/1  "-A*H_dr*exp()*(-Alhpa)"
  Gain1/1 -> Divide/1  "(-R*T)/Ea"
  Integrator1/1 -> Gain/1, Alpha/1  "Alpha"
  Gain4/1 -> Integrator1/1
  Constant3/1 -> Math Function1/2
  Constant1/1 -> Switch/3, Switch1/3
  Divide/1 -> Math Function/1  "Ea/(-R*T)"
  Math Function/1 -> Gain2/1
  Bias3/1 -> Gain3/1
  Gain3/1 -> Switch1/2
  Q_in/1 -> Add/2

== system Sim/Element43 ==
  Q_in : Inport
  Q_out : Inport  Port=2
  Add : Sum  Inputs=++-
  Bias : Bias  Bias=1
  Bias2 : Bias  Bias=-Ts
  Bias3 : Bias  Bias=-Tl
  Bias4 : Bias  Bias=-1
  Constant : Constant  Value=cv+(H_pc/(Tl-Ts))
  Constant1 : Constant  Value=cv
  Constant2 : Constant  Value=0
  Constant3 : Constant  Value=ord
  Constant4 : Constant
  Divide : Product  Inputs=/
  Divide1 : Product  Inputs=/*
  Gain : Gain  Gain=-1
  Gain1 : Gain  Gain=(-8.314)/Ea
  Gain2 : Gain  Gain=(-1)*H_dr*A
  Gain3 : Gain  Gain=-1
  Gain4 : Gain  Gain=(-1)/H_dr
  Gain5 : Gain  Gain=1/(Tl-Ts)
  Gain6 : Gain  Gain=-1
  Integrator : Integrator  InitialCondition=T_0
  Integrator1 : Integrator
  Math Function : Math  SaturateOnIntegerOverflow=on
  Math Function1 : Math  Operator=pow  SaturateOnIntegerOverflow=on
  Product : Product
  Switch : Switch
  Switch1 : Switch  Criteria=u2 > Threshold
  Switch2 : Switch
  Switch3 : Switch  Criteria=u2 > Threshold
  Beta : Outport
  Temp : Outport  Port=2
  Alpha : Outport  Port=3
  wires:
  Q_out/1 -> Add/3
  Gain/1 -> Bias/1
  Divide1/1 -> Integrator/1  "dT/dt"
  Gain2/1 -> Product/1
  Integrator/1 -> Temp/1, Bias3/1, Bias2/1, Gain1/1  "T"
  Switch1/1 -> Divide1/1  "CON"
  Math Function1/1 -> Product/2
  Bias/1 -> Math Function1/1  "(1-Alpha)"
  Constant2/1 -> Switch2/3
  Add/1 -> Divide1/2  "CON*(dT/dt)"
  Gain5/1 -> Switch2/1, Switch2/2
  Switch2/1 -> Switch3/1, Bias4/1
  Constant/1 -> Switch/1
  Bias4/1 -> Gain6/1
  Switch/1 -> Switch1/1
  Switch3/1 -> Beta/1  "Beta"
  Gain6/1 -> Switch3/2
  Bias2/1 -> Gain5/1, Switch/2
  Constant4/1 -> Switch3/3
  Product/1 -> Add/1, Gain4/1  "-A*H_dr*exp()*(-Alhpa)"
  Gain1/1 -> Divide/1  "(-R*T)/Ea"
  Integrator1/1 -> Gain/1, Alpha/1  "Alpha"
  Gain4/1 -> Integrator1/1
  Constant3/1 -> Math Function1/2
  Constant1/1 -> Switch/3, Switch1/3
  Divide/1 -> Math Function/1  "Ea/(-R*T)"
  Math Function/1 -> Gain2/1
  Bias3/1 -> Gain3/1
  Gain3/1 -> Switch1/2
  Q_in/1 -> Add/2

== system Sim/Element44 ==
  Q_in : Inport
  Q_out : Inport  Port=2
  Add : Sum  Inputs=++-
  Bias : Bias  Bias=1
  Bias2 : Bias  Bias=-Ts
  Bias3 : Bias  Bias=-Tl
  Bias4 : Bias  Bias=-1
  Constant : Constant  Value=cv+(H_pc/(Tl-Ts))
  Constant1 : Constant  Value=cv
  Constant2 : Constant  Value=0
  Constant3 : Constant  Value=ord
  Constant4 : Constant
  Divide : Product  Inputs=/
  Divide1 : Product  Inputs=/*
  Gain : Gain  Gain=-1
  Gain1 : Gain  Gain=(-8.314)/Ea
  Gain2 : Gain  Gain=(-1)*H_dr*A
  Gain3 : Gain  Gain=-1
  Gain4 : Gain  Gain=(-1)/H_dr
  Gain5 : Gain  Gain=1/(Tl-Ts)
  Gain6 : Gain  Gain=-1
  Integrator : Integrator  InitialCondition=T_0
  Integrator1 : Integrator
  Math Function : Math  SaturateOnIntegerOverflow=on
  Math Function1 : Math  Operator=pow  SaturateOnIntegerOverflow=on
  Product : Product
  Switch : Switch
  Switch1 : Switch  Criteria=u2 > Threshold
  Switch2 : Switch
  Switch3 : Switch  Criteria=u2 > Threshold
  Beta : Outport
  Temp : Outport  Port=2
  Alpha : Outport  Port=3
  wires:
  Q_out/1 -> Add/3
  Gain/1 -> Bias/1
  Divide1/1 -> Integrator/1  "dT/dt"
  Gain2/1 -> Product/1
  Integrator/1 -> Temp/1, Bias3/1, Bias2/1, Gain1/1  "T"
  Switch1/1 -> Divide1/1  "CON"
  Math Function1/1 -> Product/2
  Bias/1 -> Math Function1/1  "(1-Alpha)"
  Constant2/1 -> Switch2/3
  Add/1 -> Divide1/2  "CON*(dT/dt)"
  Gain5/1 -> Switch2/1, Switch2/2
  Switch2/1 -> Switch3/1, Bias4/1
  Constant/1 -> Switch/1
  Bias4/1 -> Gain6/1
  Switch/1 -> Switch1/1
  Switch3/1 -> Beta/1  "Beta"
  Gain6/1 -> Switch3/2
  Bias2/1 -> Gain5/1, Switch/2
  Constant4/1 -> Switch3/3
  Product/1 -> Add/1, Gain4/1  "-A*H_dr*exp()*(-Alhpa)"
  Gain1/1 -> Divide/1  "(-R*T)/Ea"
  Integrator1/1 -> Gain/1, Alpha/1  "Alpha"
  Gain4/1 -> Integrator1/1
  Constant3/1 -> Math Function1/2
  Constant1/1 -> Switch/3, Switch1/3
  Divide/1 -> Math Function/1  "Ea/(-R*T)"
  Math Function/1 -> Gain2/1
  Bias3/1 -> Gain3/1
  Gain3/1 -> Switch1/2
  Q_in/1 -> Add/2

== system Sim/Element5 ==
  Q_in : Inport
  Q_out : Inport  Port=2
  Add : Sum  Inputs=++-
  Bias : Bias  Bias=1
  Bias2 : Bias  Bias=-Ts
  Bias3 : Bias  Bias=-Tl
  Bias4 : Bias  Bias=-1
  Constant : Constant  Value=cv+(H_pc/(Tl-Ts))
  Constant1 : Constant  Value=cv
  Constant2 : Constant  Value=0
  Constant3 : Constant  Value=ord
  Constant4 : Constant
  Divide : Product  Inputs=/
  Divide1 : Product  Inputs=/*
  Gain : Gain  Gain=-1
  Gain1 : Gain  Gain=(-8.314)/Ea
  Gain2 : Gain  Gain=(-1)*H_dr*A
  Gain3 : Gain  Gain=-1
  Gain4 : Gain  Gain=(-1)/H_dr
  Gain5 : Gain  Gain=1/(Tl-Ts)
  Gain6 : Gain  Gain=-1
  Integrator : Integrator  InitialCondition=T_0
  Integrator1 : Integrator
  Math Function : Math  SaturateOnIntegerOverflow=on
  Math Function1 : Math  Operator=pow  SaturateOnIntegerOverflow=on
  Product : Product
  Switch : Switch
  Switch1 : Switch  Criteria=u2 > Threshold
  Switch2 : Switch
  Switch3 : Switch  Criteria=u2 > Threshold
  Beta : Outport
  Temp : Outport  Port=2
  Alpha : Outport  Port=3
  wires:
  Q_out/1 -> Add/3
  Gain/1 -> Bias/1
  Divide1/1 -> Integrator/1  "dT/dt"
  Gain2/1 -> Product/1
  Integrator/1 -> Temp/1, Bias3/1, Bias2/1, Gain1/1  "T"
  Switch1/1 -> Divide1/1  "CON"
  Math Function1/1 -> Product/2
  Bias/1 -> Math Function1/1  "(1-Alpha)"
  Constant2/1 -> Switch2/3
  Add/1 -> Divide1/2  "CON*(dT/dt)"
  Gain5/1 -> Switch2/1, Switch2/2
  Switch2/1 -> Switch3/1, Bias4/1
  Constant/1 -> Switch/1
  Bias4/1 -> Gain6/1
  Switch/1 -> Switch1/1
  Switch3/1 -> Beta/1  "Beta"
  Gain6/1 -> Switch3/2
  Bias2/1 -> Gain5/1, Switch/2
  Constant4/1 -> Switch3/3
  Product/1 -> Add/1, Gain4/1  "-A*H_dr*exp()*(-Alhpa)"
  Gain1/1 -> Divide/1  "(-R*T)/Ea"
  Integrator1/1 -> Gain/1, Alpha/1  "Alpha"
  Gain4/1 -> Integrator1/1
  Constant3/1 -> Math Function1/2
  Constant1/1 -> Switch/3, Switch1/3
  Divide/1 -> Math Function/1  "Ea/(-R*T)"
  Math Function/1 -> Gain2/1
  Bias3/1 -> Gain3/1
  Gain3/1 -> Switch1/2
  Q_in/1 -> Add/2

== system Sim/Element6 ==
  Q_in : Inport
  Q_out : Inport  Port=2
  Add : Sum  Inputs=++-
  Bias : Bias  Bias=1
  Bias2 : Bias  Bias=-Ts
  Bias3 : Bias  Bias=-Tl
  Bias4 : Bias  Bias=-1
  Constant : Constant  Value=cv+(H_pc/(Tl-Ts))
  Constant1 : Constant  Value=cv
  Constant2 : Constant  Value=0
  Constant3 : Constant  Value=ord
  Constant4 : Constant
  Divide : Product  Inputs=/
  Divide1 : Product  Inputs=/*
  Gain : Gain  Gain=-1
  Gain1 : Gain  Gain=(-8.314)/Ea
  Gain2 : Gain  Gain=(-1)*H_dr*A
  Gain3 : Gain  Gain=-1
  Gain4 : Gain  Gain=(-1)/H_dr
  Gain5 : Gain  Gain=1/(Tl-Ts)
  Gain6 : Gain  Gain=-1
  Integrator : Integrator  InitialCondition=T_0
  Integrator1 : Integrator
  Math Function : Math  SaturateOnIntegerOverflow=on
  Math Function1 : Math  Operator=pow  SaturateOnIntegerOverflow=on
  Product : Product
  Switch : Switch
  Switch1 : Switch  Criteria=u2 > Threshold
  Switch2 : Switch
  Switch3 : Switch  Criteria=u2 > Threshold
  Beta : Outport
  Temp : Outport  Port=2
  Alpha : Outport  Port=3
  wires:
  Q_out/1 -> Add/3
  Gain/1 -> Bias/1
  Divide1/1 -> Integrator/1  "dT/dt"
  Gain2/1 -> Product/1
  Integrator/1 -> Temp/1, Bias3/1, Bias2/1, Gain1/1  "T"
  Switch1/1 -> Divide1/1  "CON"
  Math Function1/1 -> Product/2
  Bias/1 -> Math Function1/1  "(1-Alpha)"
  Constant2/1 -> Switch2/3
  Add/1 -> Divide1/2  "CON*(dT/dt)"
  Gain5/1 -> Switch2/1, Switch2/2
  Switch2/1 -> Switch3/1, Bias4/1
  Constant/1 -> Switch/1
  Bias4/1 -> Gain6/1
  Switch/1 -> Switch1/1
  Switch3/1 -> Beta/1  "Beta"
  Gain6/1 -> Switch3/2
  Bias2/1 -> Gain5/1, Switch/2
  Constant4/1 -> Switch3/3
  Product/1 -> Add/1, Gain4/1  "-A*H_dr*exp()*(-Alhpa)"
  Gain1/1 -> Divide/1  "(-R*T)/Ea"
  Integrator1/1 -> Gain/1, Alpha/1  "Alpha"
  Gain4/1 -> Integrator1/1
  Constant3/1 -> Math Function1/2
  Constant1/1 -> Switch/3, Switch1/3
  Divide/1 -> Math Function/1  "Ea/(-R*T)"
  Math Function/1 -> Gain2/1
  Bias3/1 -> Gain3/1
  Gain3/1 -> Switch1/2
  Q_in/1 -> Add/2

== system Sim/Element7 ==
  Q_in : Inport
  Q_out : Inport  Port=2
  Add : Sum  Inputs=++-
  Bias : Bias  Bias=1
  Bias2 : Bias  Bias=-Ts
  Bias3 : Bias  Bias=-Tl
  Bias4 : Bias  Bias=-1
  Constant : Constant  Value=cv+(H_pc/(Tl-Ts))
  Constant1 : Constant  Value=cv
  Constant2 : Constant  Value=0
  Constant3 : Constant  Value=ord
  Constant4 : Constant
  Divide : Product  Inputs=/
  Divide1 : Product  Inputs=/*
  Gain : Gain  Gain=-1
  Gain1 : Gain  Gain=(-8.314)/Ea
  Gain2 : Gain  Gain=(-1)*H_dr*A
  Gain3 : Gain  Gain=-1
  Gain4 : Gain  Gain=(-1)/H_dr
  Gain5 : Gain  Gain=1/(Tl-Ts)
  Gain6 : Gain  Gain=-1
  Integrator : Integrator  InitialCondition=T_0
  Integrator1 : Integrator
  Math Function : Math  SaturateOnIntegerOverflow=on
  Math Function1 : Math  Operator=pow  SaturateOnIntegerOverflow=on
  Product : Product
  Switch : Switch
  Switch1 : Switch  Criteria=u2 > Threshold
  Switch2 : Switch
  Switch3 : Switch  Criteria=u2 > Threshold
  Beta : Outport
  Temp : Outport  Port=2
  Alpha : Outport  Port=3
  wires:
  Q_out/1 -> Add/3
  Gain/1 -> Bias/1
  Divide1/1 -> Integrator/1  "dT/dt"
  Gain2/1 -> Product/1
  Integrator/1 -> Temp/1, Bias3/1, Bias2/1, Gain1/1  "T"
  Switch1/1 -> Divide1/1  "CON"
  Math Function1/1 -> Product/2
  Bias/1 -> Math Function1/1  "(1-Alpha)"
  Constant2/1 -> Switch2/3
  Add/1 -> Divide1/2  "CON*(dT/dt)"
  Gain5/1 -> Switch2/1, Switch2/2
  Switch2/1 -> Switch3/1, Bias4/1
  Constant/1 -> Switch/1
  Bias4/1 -> Gain6/1
  Switch/1 -> Switch1/1
  Switch3/1 -> Beta/1  "Beta"
  Gain6/1 -> Switch3/2
  Bias2/1 -> Gain5/1, Switch/2
  Constant4/1 -> Switch3/3
  Product/1 -> Add/1, Gain4/1  "-A*H_dr*exp()*(-Alhpa)"
  Gain1/1 -> Divide/1  "(-R*T)/Ea"
  Integrator1/1 -> Gain/1, Alpha/1  "Alpha"
  Gain4/1 -> Integrator1/1
  Constant3/1 -> Math Function1/2
  Constant1/1 -> Switch/3, Switch1/3
  Divide/1 -> Math Function/1  "Ea/(-R*T)"
  Math Function/1 -> Gain2/1
  Bias3/1 -> Gain3/1
  Gain3/1 -> Switch1/2
  Q_in/1 -> Add/2

== system Sim/Element8 ==
  Q_in : Inport
  Q_out : Inport  Port=2
  Add : Sum  Inputs=++-
  Bias : Bias  Bias=1
  Bias2 : Bias  Bias=-Ts
  Bias3 : Bias  Bias=-Tl
  Bias4 : Bias  Bias=-1
  Constant : Constant  Value=cv+(H_pc/(Tl-Ts))
  Constant1 : Constant  Value=cv
  Constant2 : Constant  Value=0
  Constant3 : Constant  Value=ord
  Constant4 : Constant
  Divide : Product  Inputs=/
  Divide1 : Product  Inputs=/*
  Gain : Gain  Gain=-1
  Gain1 : Gain  Gain=(-8.314)/Ea
  Gain2 : Gain  Gain=(-1)*H_dr*A
  Gain3 : Gain  Gain=-1
  Gain4 : Gain  Gain=(-1)/H_dr
  Gain5 : Gain  Gain=1/(Tl-Ts)
  Gain6 : Gain  Gain=-1
  Integrator : Integrator  InitialCondition=T_0
  Integrator1 : Integrator
  Math Function : Math  SaturateOnIntegerOverflow=on
  Math Function1 : Math  Operator=pow  SaturateOnIntegerOverflow=on
  Product : Product
  Switch : Switch
  Switch1 : Switch  Criteria=u2 > Threshold
  Switch2 : Switch
  Switch3 : Switch  Criteria=u2 > Threshold
  Beta : Outport
  Temp : Outport  Port=2
  Alpha : Outport  Port=3
  wires:
  Q_out/1 -> Add/3
  Gain/1 -> Bias/1
  Divide1/1 -> Integrator/1  "dT/dt"
  Gain2/1 -> Product/1
  Integrator/1 -> Temp/1, Bias3/1, Bias2/1, Gain1/1  "T"
  Switch1/1 -> Divide1/1  "CON"
  Math Function1/1 -> Product/2
  Bias/1 -> Math Function1/1  "(1-Alpha)"
  Constant2/1 -> Switch2/3
  Add/1 -> Divide1/2  "CON*(dT/dt)"
  Gain5/1 -> Switch2/1, Switch2/2
  Switch2/1 -> Switch3/1, Bias4/1
  Constant/1 -> Switch/1
  Bias4/1 -> Gain6/1
  Switch/1 -> Switch1/1
  Switch3/1 -> Beta/1  "Beta"
  Gain6/1 -> Switch3/2
  Bias2/1 -> Gain5/1, Switch/2
  Constant4/1 -> Switch3/3
  Product/1 -> Add/1, Gain4/1  "-A*H_dr*exp()*(-Alhpa)"
  Gain1/1 -> Divide/1  "(-R*T)/Ea"
  Integrator1/1 -> Gain/1, Alpha/1  "Alpha"
  Gain4/1 -> Integrator1/1
  Constant3/1 -> Math Function1/2
  Constant1/1 -> Switch/3, Switch1/3
  Divide/1 -> Math Function/1  "Ea/(-R*T)"
  Math Function/1 -> Gain2/1
  Bias3/1 -> Gain3/1
  Gain3/1 -> Switch1/2
  Q_in/1 -> Add/2

== system Sim/Element9 ==
  Q_in : Inport
  Q_out : Inport  Port=2
  Add : Sum  Inputs=++-
  Bias : Bias  Bias=1
  Bias2 : Bias  Bias=-Ts
  Bias3 : Bias  Bias=-Tl
  Bias4 : Bias  Bias=-1
  Constant : Constant  Value=cv+(H_pc/(Tl-Ts))
  Constant1 : Constant  Value=cv
  Constant2 : Constant  Value=0
  Constant3 : Constant  Value=ord
  Constant4 : Constant
  Divide : Product  Inputs=/
  Divide1 : Product  Inputs=/*
  Gain : Gain  Gain=-1
  Gain1 : Gain  Gain=(-8.314)/Ea
  Gain2 : Gain  Gain=(-1)*H_dr*A
  Gain3 : Gain  Gain=-1
  Gain4 : Gain  Gain=(-1)/H_dr
  Gain5 : Gain  Gain=1/(Tl-Ts)
  Gain6 : Gain  Gain=-1
  Integrator : Integrator  InitialCondition=T_0
  Integrator1 : Integrator
  Math Function : Math  SaturateOnIntegerOverflow=on
  Math Function1 : Math  Operator=pow  SaturateOnIntegerOverflow=on
  Product : Product
  Switch : Switch
  Switch1 : Switch  Criteria=u2 > Threshold
  Switch2 : Switch
  Switch3 : Switch  Criteria=u2 > Threshold
  Beta : Outport
  Temp : Outport  Port=2
  Alpha : Outport  Port=3
  wires:
  Q_out/1 -> Add/3
  Gain/1 -> Bias/1
  Divide1/1 -> Integrator/1  "dT/dt"
  Gain2/1 -> Product/1
  Integrator/1 -> Temp/1, Bias3/1, Bias2/1, Gain1/1  "T"
  Switch1/1 -> Divide1/1  "CON"
  Math Function1/1 -> Product/2
  Bias/1 -> Math Function1/1  "(1-Alpha)"
  Constant2/1 -> Switch2/3
  Add/1 -> Divide1/2  "CON*(dT/dt)"
  Gain5/1 -> Switch2/1, Switch2/2
  Switch2/1 -> Switch3/1, Bias4/1
  Constant/1 -> Switch/1
  Bias4/1 -> Gain6/1
  Switch/1 -> Switch1/1
  Switch3/1 -> Beta/1  "Beta"
  Gain6/1 -> Switch3/2
  Bias2/1 -> Gain5/1, Switch/2
  Constant4/1 -> Switch3/3
  Product/1 -> Add/1, Gain4/1  "-A*H_dr*exp()*(-Alhpa)"
  Gain1/1 -> Divide/1  "(-R*T)/Ea"
  Integrator1/1 -> Gain/1, Alpha/1  "Alpha"
  Gain4/1 -> Integrator1/1
  Constant3/1 -> Math Function1/2
  Constant1/1 -> Switch/3, Switch1/3
  Divide/1 -> Math Function/1  "Ea/(-R*T)"
  Math Function/1 -> Gain2/1
  Bias3/1 -> Gain3/1
  Gain3/1 -> Switch1/2
  Q_in/1 -> Add/2

== system Sim/Heat treansfer ==
  Temp(+) : Inport
  Temp(-) : Inport  Port=2
  Gain14 : Gain  Gain=lamda/detaX/detaX
  Subtract : Sum  Inputs=+-
  Q[W/m3] : Outport
  wires:
  Temp(-)/1 -> Subtract/2
  Temp(+)/1 -> Subtract/1
  Subtract/1 -> Gain14/1  "Temp difference"
  Gain14/1 -> Q[W/m3]/1

== system Sim/Heat treansfer1 ==
  Temp(+) : Inport
  Temp(-) : Inport  Port=2
  Gain14 : Gain  Gain=lamda/detaX/detaX
  Subtract : Sum  Inputs=+-
  Q[W/m3] : Outport
  wires:
  Temp(-)/1 -> Subtract/2
  Temp(+)/1 -> Subtract/1
  Subtract/1 -> Gain14/1  "Temp difference"
  Gain14/1 -> Q[W/m3]/1

== system Sim/Heat treansfer10 ==
  Temp(+) : Inport
  Temp(-) : Inport  Port=2
  Gain14 : Gain  Gain=lamda/detaX/detaX
  Subtract : Sum  Inputs=+-
  Q[W/m3] : Outport
  wires:
  Temp(-)/1 -> Subtract/2
  Temp(+)/1 -> Subtract/1
  Subtract/1 -> Gain14/1  "Temp difference"
  Gain14/1 -> Q[W/m3]/1

== system Sim/Heat treansfer11 ==
  Temp(+) : Inport
  Temp(-) : Inport  Port=2
  Gain14 : Gain  Gain=lamda/detaX/detaX
  Subtract : Sum  Inputs=+-
  Q[W/m3] : Outport
  wires:
  Temp(-)/1 -> Subtract/2
  Temp(+)/1 -> Subtract/1
  Subtract/1 -> Gain14/1  "Temp difference"
  Gain14/1 -> Q[W/m3]/1

== system Sim/Heat treansfer12 ==
  Temp(+) : Inport
  Temp(-) : Inport  Port=2
  Gain14 : Gain  Gain=lamda/detaX/detaX
  Subtract : Sum  Inputs=+-
  Q[W/m3] : Outport
  wires:
  Temp(-)/1 -> Subtract/2
  Temp(+)/1 -> Subtract/1
  Subtract/1 -> Gain14/1  "Temp difference"
  Gain14/1 -> Q[W/m3]/1
